simulink subsystem "full_controller_feedbackLinearization"  (R2022a)
settings: Solver=VariableStepAuto  StartTime=0.0  StopTime=10.0  RelTol=1e-3
settings Model: Creator=Philipp  LastModifiedBy=Philipp
settings DebuggingCC: UnconnectedInputMsg=warning  UnconnectedOutputMsg=warning  UnconnectedLineMsg=warning
settings RTWCC: DLArmComputeVersion=19.05

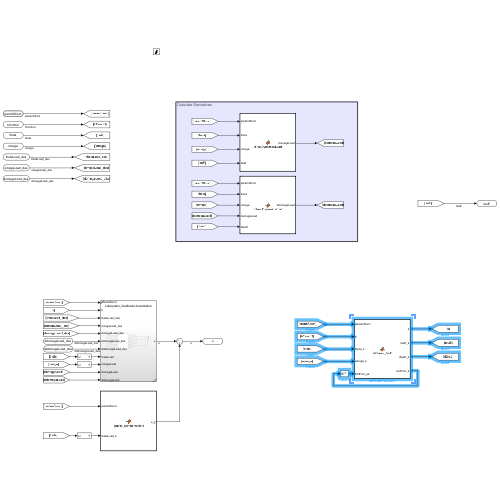
[thumbnail: Simulink's stored preview of the top-level diagram]
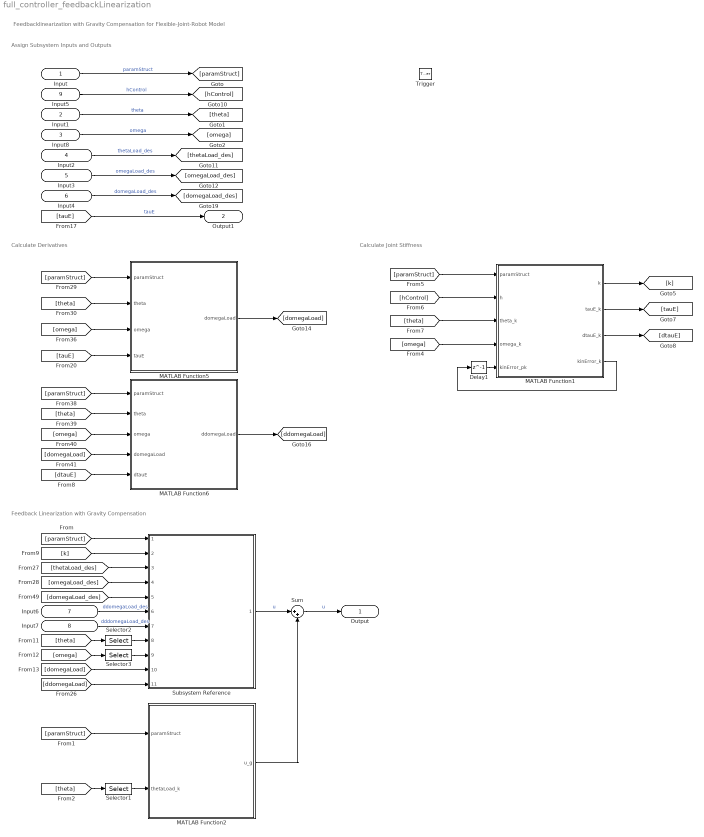
== system full_controller_feedbackLinearization ==
  note: Calculate Joint Stiffness
  note: Feedback Linearization with Gravity Compensation
  note: Calculate Derivatives
  note: Assign Subsystem Inputs and Outputs
  note: Feedbacklinearization with Gravity Compensation for Flexible-Joint-Robot Model
  Input : Inport  OutDataTypeStr=Bus: main_bus
  Input1 : Inport  Port=2
  Input8 : Inport  Port=3
  Input2 : Inport  Port=4
  Input3 : Inport  Port=5
  Input4 : Inport  Port=6
  Input6 : Inport  Port=7
  Input7 : Inport  Port=8
  Input5 : Inport  Port=9
  Trigger : TriggerPort  VariantControl=(inherit)
  Delay1 : Delay  DelayLength=1
  MATLAB Function1 : MATLAB Function  TreatAsAtomicUnit=on
  MATLAB Function2 : MATLAB Function  TreatAsAtomicUnit=on
  MATLAB Function5 : MATLAB Function  TreatAsAtomicUnit=on
  MATLAB Function6 : MATLAB Function  TreatAsAtomicUnit=on
  Selector1 : Selector  InputPortWidth=6  IndexOptions=Index vector (dialog)  Indices=1:3  OutputSizes=1
  Selector2 : Selector  InputPortWidth=6  IndexOptions=Index vector (dialog)  Indices=1:3  OutputSizes=1
  Selector3 : Selector  InputPortWidth=6  IndexOptions=Index vector (dialog)  Indices=1:3  OutputSizes=1
  Subsystem Reference : Subsystem  ReferencedSubsystem=subsystem_feedbackLinearization
  Sum : Sum  Inputs=|++
  Output : Outport
  Output1 : Outport  Port=2
  wires:
  Input/1 -> [paramStruct]  "paramStruct"
  Input1/1 -> [theta]  "theta"
  MATLAB Function1/2(tauE_k) -> [tauE]
  MATLAB Function1/3(dtauE_k) -> [dtauE]
  Input5/1 -> [hControl]  "hControl"
  MATLAB Function1/1(k) -> [k]
  Input2/1 -> [thetaLoad_des]  "thetaLoad_des"
  Input3/1 -> [omegaLoad_des]  "omegaLoad_des"
  [paramStruct] -> MATLAB Function5/1(paramStruct)
  [theta] -> MATLAB Function5/2(theta)
  [omega] -> MATLAB Function5/3(omega)
  MATLAB Function5/1(domegaLoad) -> [domegaLoad]
  [paramStruct] -> MATLAB Function6/1(paramStruct)
  [theta] -> MATLAB Function6/2(theta)
  [omega] -> MATLAB Function6/3(omega)
  [domegaLoad] -> MATLAB Function6/4(domegaLoad)
  Input4/1 -> [domegaLoad_des]  "domegaLoad_des"
  [paramStruct] -> Subsystem Reference/1
  [thetaLoad_des] -> Subsystem Reference/3
  [omegaLoad_des] -> Subsystem Reference/4
  [domegaLoad_des] -> Subsystem Reference/5
  [theta] -> Selector2/1
  [omega] -> Selector3/1
  [domegaLoad] -> Subsystem Reference/10
  [ddomegaLoad] -> Subsystem Reference/11
  Input6/1 -> Subsystem Reference/6  "ddomegaLoad_des"
  Input7/1 -> Subsystem Reference/7  "dddomegaLoad_des"
  MATLAB Function6/1(ddomegaLoad) -> [ddomegaLoad]
  Input8/1 -> [omega]  "omega"
  [paramStruct] -> MATLAB Function1/1(paramStruct)
  [hControl] -> MATLAB Function1/2(h)
  [theta] -> MATLAB Function1/3(theta_k)
  [omega] -> MATLAB Function1/4(omega_k)
  Delay1/1 -> MATLAB Function1/5(kinError_pk)
  MATLAB Function1/4(kinError_k) -> Delay1/1
  [tauE] -> MATLAB Function5/4(tauE)
  [dtauE] -> MATLAB Function6/5(dtauE)
  Selector2/1 -> Subsystem Reference/8
  Selector3/1 -> Subsystem Reference/9
  [k] -> Subsystem Reference/2
  [tauE] -> Output1/1  "tauE"
  Sum/1 -> Output/1  "u"
  Subsystem Reference/1 -> Sum/1  "u"
  MATLAB Function2/1(u_g) -> Sum/2
  [paramStruct] -> MATLAB Function2/1(paramStruct)
  [theta] -> Selector1/1
  Selector1/1 -> MATLAB Function2/2(thetaLoad_k)

== matlab function full_controller_feedbackLinearization/MATLAB Function2 ==
  data: u_g output; paramStruct input; thetaLoad_k input
function u_g = gravity_compensation(paramStruct, thetaLoad_k)

g = paramStruct.robot.g;
r_P1P2 = paramStruct.robot.r_P1P2;
r_P2P3 = paramStruct.robot.r_P2P3;
r_P3P4 = paramStruct.robot.r_P3P4;
baseParam = paramStruct.robot.baseParam;

u_g = gravityCompensation_fun(g, r_P1P2, r_P2P3, r_P3P4, baseParam, thetaLoad_k);

== matlab function full_controller_feedbackLinearization/MATLAB Function1 ==
  data: k output; tauE_k output; dtauE_k output; paramStruct input; h input; theta_k input; omega_k input; kinError_pk input; kinError_k output size=3
function [k, tauE_k, dtauE_k, kinError_k] = stiffness_tauE(paramStruct, h, theta_k, omega_k, kinError_pk)

% Convert to deg
thetaDeg_k = theta_k .* (180/pi);
omegaDeg_k = omega_k .* (180/pi);

% Calculate kinematic error
%kinErrorDeg_k = kinError_fun(paramStruct, thetaDeg_k(4:6);
kinErrorDeg_k = zeros(3,1); % Do not consider in model because it results in sigularities for numerical integration
%dkinErrorDeg_k = discreteDiff_fun(h, kinErrorDeg_k, kinError_pk);
dkinErrorDeg_k = zeros(3,1); % Do not consider in model because it results in sigularities for numerical integration

% Calculate stiffness
[thetaDiffE_k, omegaDiffE_k] = compKinError_fun(thetaDeg_k, omegaDeg_k, kinErrorDeg_k, dkinErrorDeg_k);
kDeg = stiffness_fun(paramStruct, thetaDiffE_k);

% Calculate stiffness torque
[tauE_k, dtauE_k] = stiffnessTorque_fun(kDeg, thetaDiffE_k, omegaDiffE_k);

% Convert to rad
kinError_k = kinErrorDeg_k .* (pi/180);
k = kDeg .* (180/pi);

== matlab function full_controller_feedbackLinearization/MATLAB Function5 ==
  data: paramStruct input; theta input; domegaLoad output; omega input; tauE input
function domegaLoad = directDynamicsLoad(paramStruct, theta, omega, tauE)

g = paramStruct.robot.g;
r_P1P2 = paramStruct.robot.r_P1P2;
r_P2P3 = paramStruct.robot.r_P2P3;
r_P3P4 = paramStruct.robot.r_P3P4;
baseParam = paramStruct.robot.baseParam;

domegaLoad = directDynamicsLoad_reduced_fun(g, r_P1P2, r_P2P3, r_P3P4, baseParam, theta(1:3), omega(1:3), tauE);

== matlab function full_controller_feedbackLinearization/MATLAB Function6 ==
  data: paramStruct input; theta input; ddomegaLoad output; omega input; domegaLoad input; dtauE input
function ddomegaLoad = ddirectDynamicsLoad(paramStruct, theta, omega, domegaLoad, dtauE)

g = paramStruct.robot.g;
r_P1P2 = paramStruct.robot.r_P1P2;
r_P2P3 = paramStruct.robot.r_P2P3;
r_P3P4 = paramStruct.robot.r_P3P4;
baseParam = paramStruct.robot.baseParam;

ddomegaLoad = ddirectDynamicsLoad_reduced_fun(g, r_P1P2, r_P2P3, r_P3P4, baseParam, theta(1:3), omega(1:3), domegaLoad, dtauE);
